simulink model "guangfu"  (R2014b)
settings: Solver=ode45  StartTime=0.0  StopTime=10.0  RelTol=1e-3
undefined symbols (not defined in the file or in its folder): K
settings Model: Creator=DELL  LastModifiedBy=dell

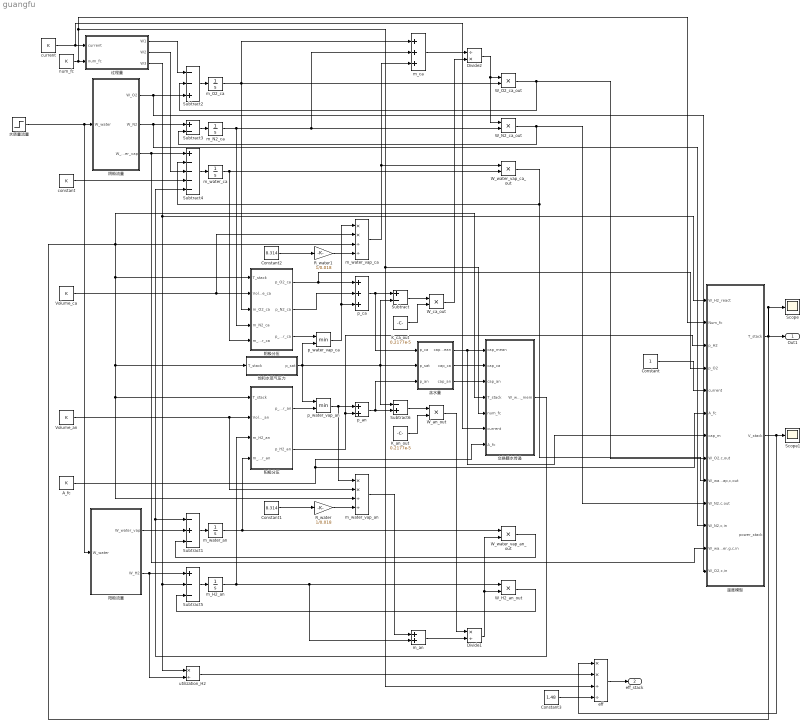
== system guangfu ==
  A_fc : Constant  Value=K
  Constant : Constant
  Constant1 : Constant  Value=8.314
  Constant2 : Constant  Value=8.314
  Constant3 : Constant  Value=1.48
  Divide1 : Product  Inputs=*/
  Divide2 : Product  Inputs=/*
  K_an_out : Constant  Value=0.2177e-5
  K_ca_out : Constant  Value=0.2177e-5
  R_water : Gain  Gain=1/0.018
  R_water1 : Gain  Gain=1/0.018
  Scope : Scope
  Scope1 : Scope
  Subtract : Sum  Inputs=+-
  Subtract1 : Sum  Inputs=-+-
  Subtract2 : Sum  Inputs=--+
  Subtract3 : Sum  Inputs=+-
  Subtract4 : Sum  Inputs=+----
  Subtract5 : Sum  Inputs=+--
  Subtract6 : Sum  Inputs=-+
  Volume_an : Constant  Value=K
  Volume_ca : Constant  Value=K
  W_H2_an_out : Product
  W_N2_ca_out : Product
  W_O2_ca_out : Product
  W_an_out : Product
  W_ca_out : Product
  W_water_vap_an_out : Product
  W_water_vap_ca_out : Product
  constant : Constant  Value=K
  current : Constant  Value=K
  eff : Product  Inputs=**//
  m_H2_an : Integrator
  m_N2_ca : Integrator
  m_O2_ca : Integrator
  m_an : Sum
  m_ca : Sum  Inputs=+++
  m_water_an : Integrator
  m_water_ca : Integrator
  m_water_vap_an : Product  Inputs=**//
  m_water_vap_ca : Product  Inputs=**//
  num_fc : Constant  Value=K
  p_an : Sum
  p_ca : Sum  Inputs=3
  p_water_vap_an : MinMax  Inputs=2
  p_water_vap_ca : MinMax  Inputs=2
  utilization_H2 : Product  Inputs=*/
  交换膜水传递 : Subsystem  TreatAsAtomicUnit=on
  含水量 : Subsystem
  水质量流量 : Step  SampleTime=0
  温度模型 : Subsystem
  过程量 : Subsystem
  阳极分压 : Subsystem
  阳极流量 : Subsystem
  阴极分压 : Subsystem
  阴极流量 : Subsystem  TreatAsAtomicUnit=on
  饱和水蒸气压力 : Subsystem
  Out1 : Outport
  eff_stack : Outport  Port=2
  wires:
  温度模型/2(V_stack) -> Scope1/1, eff/1
  Constant/1 -> 温度模型/5(current)
  Volume_ca/1 -> m_water_vap_ca/2, 阴极分压/2(Volume_ca)
  阴极分压/3(p_water_ca) -> p_water_vap_ca/1
  饱和水蒸气压力/1(p_sat) -> p_water_vap_an/1, Subtract/2, 含水量/2(p_sat), Subtract6/1, p_water_vap_ca/2
  p_water_vap_ca/1 -> m_water_vap_ca/1, p_ca/3
  p_ca/1 -> Subtract/1, 含水量/1(p_ca)
  Subtract/1 -> W_ca_out/1
  K_ca_out/1 -> W_ca_out/2
  阴极流量/1(W_O2) -> 温度模型/13(W_O2,c,in), Subtract2/3
  过程量/3(W3) -> utilization_H2/1, Subtract5/2, 温度模型/1(W_H2_react)
  过程量/1(W1) -> Subtract2/1
  Subtract2/1 -> m_O2_ca/1
  阴极流量/2(W_N2) -> 温度模型/11(W_N2,c,in), Subtract3/1
  Subtract3/1 -> m_N2_ca/1
  阴极流量/3(W_water_vap) -> 温度模型/12(W_water,g,c,in), Subtract4/1
  Subtract4/1 -> m_water_ca/1
  过程量/2(W2) -> Subtract4/3
  constant/1 -> Subtract4/4
  m_O2_ca/1 -> W_O2_ca_out/2, m_ca/1, 阴极分压/3(m_O2_ca)
  m_N2_ca/1 -> W_N2_ca_out/2, m_ca/2, 阴极分压/4(m_N2_ca)
  温度模型/1(T_stack) -> m_water_vap_an/3, 阳极分压/1(T_stack), 饱和水蒸气压力/1(T_stack), 阴极分压/1(T_stack), 交换膜水传递/4(T_stack), m_water_vap_ca/3, Scope/1, Out1/1
  m_water_vap_ca/1 -> m_ca/3, W_water_vap_ca_out/1
  m_water_ca/1 -> W_water_vap_ca_out/2, 阴极分压/5(m_water_ca)
  Constant2/1 -> R_water1/1
  R_water1/1 -> m_water_vap_ca/4
  阴极分压/2(p_N2_ca) -> p_ca/2
  m_ca/1 -> Divide2/1
  W_ca_out/1 -> Divide2/2
  Divide2/1 -> W_N2_ca_out/1, W_O2_ca_out/1
  W_O2_ca_out/1 -> 温度模型/8(W_O2,c,out), Subtract2/2
  W_N2_ca_out/1 -> 温度模型/10(W_N2,c,out), Subtract3/2
  W_water_vap_ca_out/1 -> Subtract4/2, 温度模型/9(W_water,vap,c,out)
  交换膜水传递/1(W_water_mem) -> Subtract4/5, Subtract1/1
  水质量流量/1 -> 阳极流量/1(W_water), 阴极流量/1(W_water)
  阳极流量/2(W_H2) -> utilization_H2/2, Subtract5/1
  Subtract5/1 -> m_H2_an/1
  Subtract1/1 -> m_water_an/1
  阳极分压/1(p_water_an) -> p_water_vap_an/2
  p_water_vap_an/1 -> p_an/1, m_water_vap_an/1
  阳极分压/2(p_H2_an) -> 温度模型/3(p_H2), p_an/2
  Constant1/1 -> R_water/1
  R_water/1 -> m_water_vap_an/4
  Volume_an/1 -> 阳极分压/2(Volume_an), m_water_vap_an/2
  Subtract6/1 -> W_an_out/1
  K_an_out/1 -> W_an_out/2
  m_water_vap_an/1 -> m_an/1
  m_H2_an/1 -> 阳极分压/3(m_H2_an), W_H2_an_out/1, m_an/2
  W_an_out/1 -> Divide1/1
  m_an/1 -> Divide1/2
  m_water_an/1 -> 阳极分压/4(m_water_an), W_water_vap_an_out/1
  Divide1/1 -> W_H2_an_out/2, W_water_vap_an_out/2
  阳极流量/1(W_water_vap) -> Subtract1/2
  W_water_vap_an_out/1 -> Subtract1/3
  W_H2_an_out/1 -> Subtract5/3
  p_an/1 -> Subtract6/2, 含水量/3(p_an)
  含水量/1(cap_mean) -> 温度模型/7(cap_m), 交换膜水传递/1(cap_mean)
  current/1 -> 交换膜水传递/6(current), 过程量/1(current)
  含水量/2(cap_ca) -> 交换膜水传递/2(cap_ca)
  含水量/3(cap_an) -> 交换膜水传递/3(cap_an)
  A_fc/1 -> 温度模型/6(A_fc), 交换膜水传递/7(A_fc)
  utilization_H2/1 -> eff/2
  num_fc/1 -> 温度模型/2(Num_fc), eff/3, 交换膜水传递/5(num_fc), 过程量/2(num_fc)
  Constant3/1 -> eff/4
  eff/1 -> eff_stack/1
  阴极分压/1(p_O2_ca) -> 温度模型/4(p_O2), p_ca/1

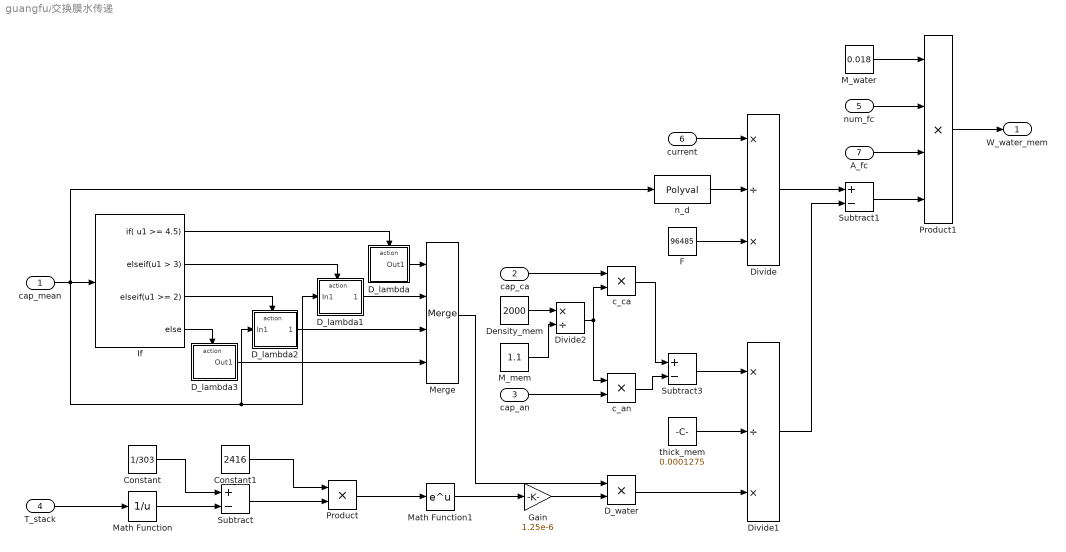
== system guangfu/交换膜水传递 ==
  cap_mean : Inport
  cap_ca : Inport  Port=2
  cap_an : Inport  Port=3
  T_stack : Inport  Port=4
  num_fc : Inport  Port=5
  current : Inport  Port=6
  A_fc : Inport  Port=7
  Constant : Constant  Value=1/303
  Constant1 : Constant  Value=2416
  D_lambda : Subsystem  TreatAsAtomicUnit=on
  D_lambda1 : Subsystem  TreatAsAtomicUnit=on
  D_lambda2 : Subsystem  TreatAsAtomicUnit=on
  D_lambda3 : Subsystem  TreatAsAtomicUnit=on
  D_water : Product
  Density_mem : Constant  Value=2000
  Divide : Product  Inputs=*/*
  Divide1 : Product  Inputs=*/*
  Divide2 : Product  Inputs=*/
  F : Constant  Value=96485
  Gain : Gain  Gain=1.25e-6
  If : If  IfExpression=u1 >= 4.5  ElseIfExpressions=u1 > 3,u1 >= 2  ZeroCross=off
  M_mem : Constant  Value=1.1
  M_water : Constant  Value=0.018
  Math Function : Math  Operator=reciprocal  SaturateOnIntegerOverflow=on
  Math Function1 : Math  SaturateOnIntegerOverflow=on
  Merge : Merge  Inputs=4
  Product : Product
  Product1 : Product  Inputs=4
  Subtract : Sum  Inputs=+-
  Subtract1 : Sum  Inputs=+-
  Subtract3 : Sum  Inputs=+-
  c_an : Product
  c_ca : Product
  n_d : Polyval  Coefs=[0.0029,0.05,-3.4e-19]
  thick_mem : Constant  Value=0.0001275
  W_water_mem : Outport
  wires:
  If/1 -> D_lambda/Action
  If/2 -> D_lambda1/Action
  If/3 -> D_lambda2/Action
  If/4 -> D_lambda3/Action
  D_lambda/1(Out1) -> Merge/1
  D_lambda1/1(Out1) -> Merge/2
  D_lambda2/1(Out1) -> Merge/3
  D_lambda3/1(Out1) -> Merge/4
  T_stack/1 -> Math Function/1
  Math Function/1 -> Subtract/2
  Constant/1 -> Subtract/1
  Subtract/1 -> Product/2
  Constant1/1 -> Product/1
  Product/1 -> Math Function1/1
  Math Function1/1 -> Gain/1
  Merge/1 -> D_water/1
  cap_mean/1 -> n_d/1, D_lambda1/1(In1), D_lambda2/1(In1), If/1
  n_d/1 -> Divide/2
  F/1 -> Divide/3
  current/1 -> Divide/1
  cap_ca/1 -> c_ca/1
  Divide/1 -> Subtract1/1
  Divide1/1 -> Subtract1/2
  D_water/1 -> Divide1/3
  thick_mem/1 -> Divide1/2
  Subtract3/1 -> Divide1/1
  Subtract1/1 -> Product1/4
  A_fc/1 -> Product1/3
  num_fc/1 -> Product1/2
  M_water/1 -> Product1/1
  Product1/1 -> W_water_mem/1
  M_mem/1 -> Divide2/2
  Density_mem/1 -> Divide2/1
  Divide2/1 -> c_an/1, c_ca/2
  c_an/1 -> Subtract3/2
  c_ca/1 -> Subtract3/1
  cap_an/1 -> c_an/2
  Gain/1 -> D_water/2

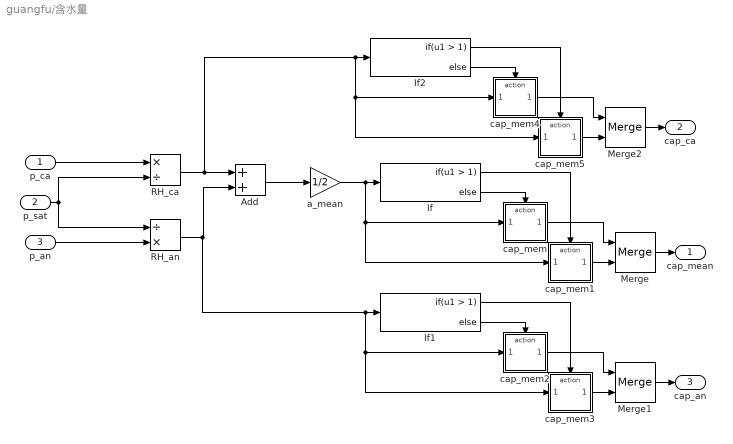
== system guangfu/含水量 ==
  p_ca : Inport
  p_sat : Inport  Port=2
  p_an : Inport  Port=3
  Add : Sum
  If : If  IfExpression=u1 > 1
  If1 : If  IfExpression=u1 > 1
  If2 : If  IfExpression=u1 > 1
  Merge : Merge
  Merge1 : Merge
  Merge2 : Merge
  RH_an : Product  Inputs=/*
  RH_ca : Product  Inputs=*/
  a_mean : Gain  Gain=1/2
  cap_mem : Subsystem  TreatAsAtomicUnit=on
  cap_mem1 : Subsystem  TreatAsAtomicUnit=on
  cap_mem2 : Subsystem  TreatAsAtomicUnit=on
  cap_mem3 : Subsystem  TreatAsAtomicUnit=on
  cap_mem4 : Subsystem  TreatAsAtomicUnit=on
  cap_mem5 : Subsystem  TreatAsAtomicUnit=on
  cap_mean : Outport
  cap_ca : Outport  Port=2
  cap_an : Outport  Port=3
  wires:
  Add/1 -> a_mean/1
  cap_mem/1(Out1) -> Merge/1
  a_mean/1 -> cap_mem1/1(In1), cap_mem/1(In1), If/1
  Merge/1 -> cap_mean/1
  If/2 -> cap_mem/Action
  p_ca/1 -> RH_ca/1
  cap_mem1/1(Out1) -> Merge/2
  If/1 -> cap_mem1/Action
  p_sat/1 -> RH_ca/2, RH_an/1
  p_an/1 -> RH_an/2
  cap_mem2/1(Out1) -> Merge1/1
  RH_an/1 -> cap_mem3/1(In1), cap_mem2/1(In1), If1/1, Add/2
  Merge1/1 -> cap_an/1
  If1/2 -> cap_mem2/Action
  cap_mem3/1(Out1) -> Merge1/2
  If1/1 -> cap_mem3/Action
  cap_mem4/1(Out1) -> Merge2/1
  RH_ca/1 -> cap_mem5/1(In1), cap_mem4/1(In1), If2/1, Add/1
  Merge2/1 -> cap_ca/1
  If2/2 -> cap_mem4/Action
  cap_mem5/1(Out1) -> Merge2/2
  If2/1 -> cap_mem5/Action

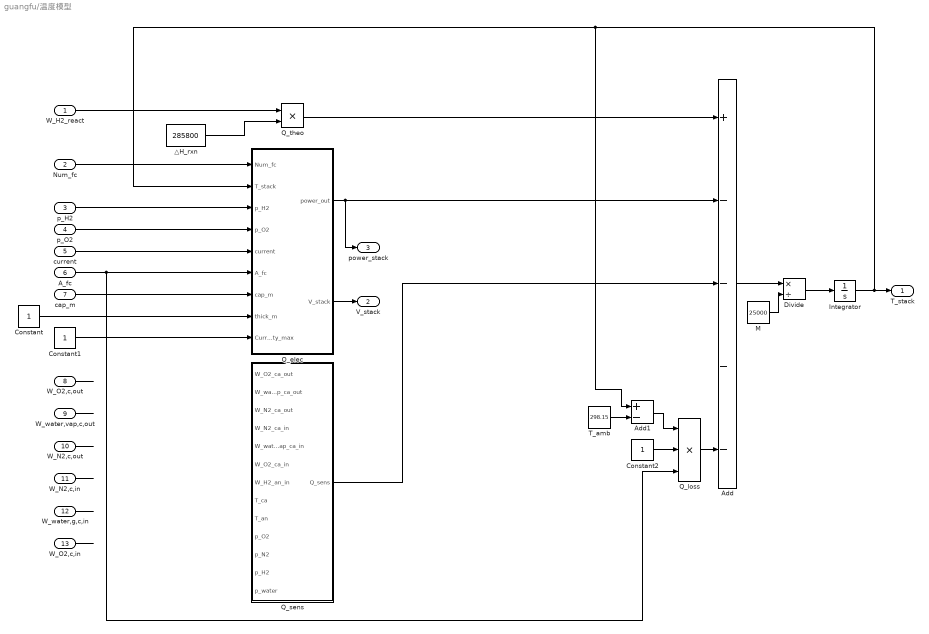
== system guangfu/温度模型 ==
  W_H2_react : Inport
  Num_fc : Inport  Port=2
  p_H2 : Inport  Port=3
  p_O2 : Inport  Port=4
  current : Inport  Port=5
  A_fc : Inport  Port=6
  cap_m : Inport  Port=7
  W_O2,c,out : Inport  Port=8
  W_water,vap,c,out : Inport  Port=9
  W_N2,c,out : Inport  Port=10
  W_N2,c,in : Inport  Port=11
  W_water,g,c,in : Inport  Port=12
  W_O2,c,in : Inport  Port=13
  Add : Sum  Inputs=+----
  Add1 : Sum  Inputs=+-
  Constant : Constant
  Constant1 : Constant
  Constant2 : Constant
  Divide : Product  Inputs=*/
  Integrator : Integrator
  M : Constant  Value=25000
  Q_elec : Subsystem
  Q_loss : Product  Inputs=3
  Q_sens : Subsystem
  Q_theo : Product
  T_amb : Constant  Value=298.15
  △H_rxn : Constant  Value=285800
  T_stack : Outport
  V_stack : Outport  Port=2
  power_stack : Outport  Port=3
  wires:
  W_H2_react/1 -> Q_theo/1
  current/1 -> Q_elec/5(current)
  p_O2/1 -> Q_elec/4(p_O2)
  p_H2/1 -> Q_elec/3(p_H2)
  W_O2,c,out/1 -> ?
  W_water,vap,c,out/1 -> ?
  W_N2,c,out/1 -> ?
  W_N2,c,in/1 -> ?
  W_water,g,c,in/1 -> ?
  W_O2,c,in/1 -> ?
  Q_elec/2(V_stack) -> V_stack/1
  △H_rxn/1 -> Q_theo/2
  Q_elec/1(power_out) -> Add/2, power_stack/1
  Q_theo/1 -> Add/1
  Q_sens/1(Q_sens) -> Add/3
  Add/1 -> Divide/1
  M/1 -> Divide/2
  Add1/1 -> Q_loss/1
  Q_loss/1 -> Add/5
  Constant2/1 -> Q_loss/2
  Divide/1 -> Integrator/1
  Integrator/1 -> Add1/1, Q_elec/2(T_stack), T_stack/1
  Num_fc/1 -> Q_elec/1(Num_fc)
  cap_m/1 -> Q_elec/7(cap_m)
  Constant/1 -> Q_elec/8(thick_m)
  T_amb/1 -> Add1/2
  A_fc/1 -> Q_loss/3, Q_elec/6(A_fc)
  Constant1/1 -> Q_elec/9(CurrentDensity_max)

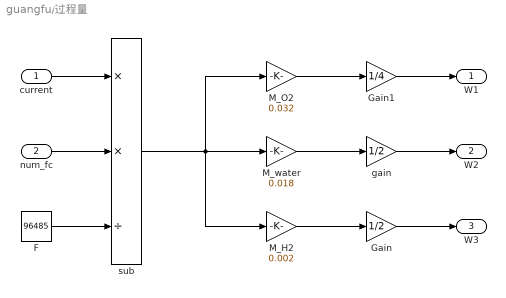
== system guangfu/过程量 ==
  current : Inport
  num_fc : Inport  Port=2
  F : Constant  Value=96485
  Gain : Gain  Gain=1/2
  Gain1 : Gain  Gain=1/4
  M_H2 : Gain  Gain=0.002
  M_O2 : Gain  Gain=0.032
  M_water : Gain  Gain=0.018
  gain : Gain  Gain=1/2
  sub : Product  Inputs=**/
  W1 : Outport
  W2 : Outport  Port=2
  W3 : Outport  Port=3
  wires:
  current/1 -> sub/1
  sub/1 -> M_water/1, M_O2/1, M_H2/1
  num_fc/1 -> sub/2
  F/1 -> sub/3
  M_H2/1 -> Gain/1
  Gain1/1 -> W1/1
  M_O2/1 -> Gain1/1
  Gain/1 -> W3/1
  M_water/1 -> gain/1
  gain/1 -> W2/1

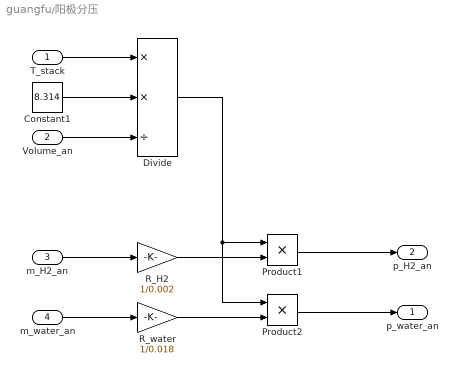
== system guangfu/阳极分压 ==
  T_stack : Inport
  Volume_an : Inport  Port=2
  m_H2_an : Inport  Port=3
  m_water_an : Inport  Port=4
  Constant1 : Constant  Value=8.314
  Divide : Product  Inputs=**/
  Product1 : Product
  Product2 : Product
  R_H2 : Gain  Gain=1/0.002
  R_water : Gain  Gain=1/0.018
  p_water_an : Outport
  p_H2_an : Outport  Port=2
  wires:
  T_stack/1 -> Divide/1
  Volume_an/1 -> Divide/3
  Constant1/1 -> Divide/2
  m_H2_an/1 -> R_H2/1
  m_water_an/1 -> R_water/1
  R_H2/1 -> Product1/2
  R_water/1 -> Product2/2
  Product1/1 -> p_H2_an/1
  Product2/1 -> p_water_an/1
  Divide/1 -> Product2/1, Product1/1

== system guangfu/阳极流量 ==
  W_water : Inport
  Constant1 : Constant
  Constant2 : Constant
  W_H2_in : Product
  W_water_in : Product
  x_H2 : Sum  Inputs=+-
  W_water_vap : Outport
  W_H2 : Outport  Port=2
  wires:
  W_water/1 -> W_water_in/1, W_H2_in/1
  ? -> W_water_in/2, x_H2/2
  Constant1/1 -> x_H2/1
  x_H2/1 -> W_H2_in/2
  W_H2_in/1 -> W_H2/1
  W_water_in/1 -> W_water_vap/1

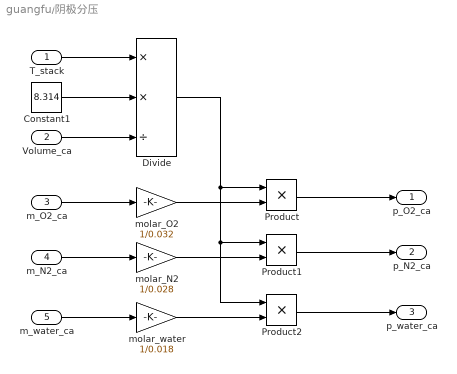
== system guangfu/阴极分压 ==
  T_stack : Inport
  Volume_ca : Inport  Port=2
  m_O2_ca : Inport  Port=3
  m_N2_ca : Inport  Port=4
  m_water_ca : Inport  Port=5
  Constant1 : Constant  Value=8.314
  Divide : Product  Inputs=**/
  Product : Product
  Product1 : Product
  Product2 : Product
  molar_N2 : Gain  Gain=1/0.028
  molar_O2 : Gain  Gain=1/0.032
  molar_water : Gain  Gain=1/0.018
  p_O2_ca : Outport
  p_N2_ca : Outport  Port=2
  p_water_ca : Outport  Port=3
  wires:
  T_stack/1 -> Divide/1
  Volume_ca/1 -> Divide/3
  Constant1/1 -> Divide/2
  m_O2_ca/1 -> molar_O2/1
  m_N2_ca/1 -> molar_N2/1
  m_water_ca/1 -> molar_water/1
  molar_O2/1 -> Product/2
  Divide/1 -> Product/1, Product1/1, Product2/1
  Product/1 -> p_O2_ca/1
  molar_N2/1 -> Product1/2
  molar_water/1 -> Product2/2
  Product1/1 -> p_N2_ca/1
  Product2/1 -> p_water_ca/1

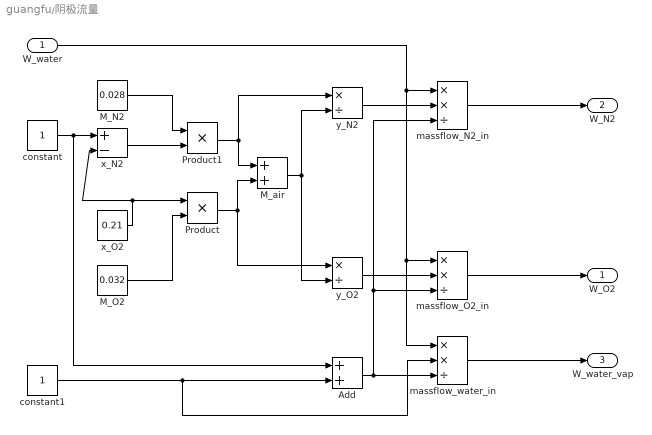
== system guangfu/阴极流量 ==
  W_water : Inport
  Add : Sum
  M_N2 : Constant  Value=0.028
  M_O2 : Constant  Value=0.032
  M_air : Sum
  Product : Product
  Product1 : Product
  constant : Constant
  constant1 : Constant
  massflow_N2_in : Product  Inputs=**/
  massflow_O2_in : Product  Inputs=**/
  massflow_water_in : Product  Inputs=**/
  x_N2 : Sum  Inputs=+-
  x_O2 : Constant  Value=0.21
  y_N2 : Product  Inputs=*/
  y_O2 : Product  Inputs=*/
  W_O2 : Outport
  W_N2 : Outport  Port=2
  W_water_vap : Outport  Port=3
  wires:
  constant/1 -> Add/1, x_N2/1
  x_O2/1 -> Product/1, x_N2/2
  M_O2/1 -> Product/2
  M_N2/1 -> Product1/1
  x_N2/1 -> Product1/2
  Product1/1 -> M_air/1, y_N2/1
  Product/1 -> M_air/2, y_O2/1
  M_air/1 -> y_O2/2, y_N2/2
  constant1/1 -> massflow_water_in/2, Add/2
  W_water/1 -> massflow_water_in/1, massflow_O2_in/1, massflow_N2_in/1
  y_N2/1 -> massflow_N2_in/2
  Add/1 -> massflow_water_in/3, massflow_N2_in/3, massflow_O2_in/3
  y_O2/1 -> massflow_O2_in/2
  massflow_N2_in/1 -> W_N2/1
  massflow_O2_in/1 -> W_O2/1
  massflow_water_in/1 -> W_water_vap/1

== system guangfu/饱和水蒸气压力 ==
  T_stack : Inport
  Constant : Constant  Value=273.15
  Math Function : Math  Operator=10^u  SaturateOnIntegerOverflow=on
  Polynomial : Polyval  Coefs=[1.4454e-7,-9.1837e-5,0.2953,-2.1794]
  T : Sum  Inputs=+-
  p_sat : Outport
  wires:
  Polynomial/1 -> Math Function/1
  T_stack/1 -> T/1
  Math Function/1 -> p_sat/1
  T/1 -> Polynomial/1
  Constant/1 -> T/2

== system guangfu/交换膜水传递/D_lambda ==
  Action Port : ActionPort  ActionType=then
  Constant : Constant  Value=1.25e-6
  Out1 : Outport
  wires:
  Constant/1 -> Out1/1

== system guangfu/交换膜水传递/D_lambda1 ==
  In1 : Inport
  Action Port : ActionPort  ActionType=elseif
  Constant : Constant  Value=3
  Constant1 : Constant  Value=1.67
  Gain : Gain  Gain=1e-6
  Product : Product
  Subtract : Sum  Inputs=+-
  Subtract1 : Sum  Inputs=+-
  Out1 : Outport
  wires:
  In1/1 -> Subtract/1
  Constant/1 -> Subtract/2, Subtract1/1
  Constant1/1 -> Product/1
  Subtract/1 -> Product/2
  Product/1 -> Subtract1/2
  Subtract1/1 -> Gain/1
  Gain/1 -> Out1/1

== system guangfu/交换膜水传递/D_lambda2 ==
  In1 : Inport
  Action Port : ActionPort  ActionType=elseif
  Add : Sum
  Constant : Constant  Value=2
  Constant1 : Constant
  Gain : Gain  Gain=1e-6
  Product : Product
  Subtract : Sum  Inputs=+-
  Out1 : Outport
  wires:
  In1/1 -> Subtract/1
  Constant/1 -> Product/2, Subtract/2
  Subtract/1 -> Product/1
  Product/1 -> Add/2
  Add/1 -> Gain/1
  Gain/1 -> Out1/1
  Constant1/1 -> Add/1

== system guangfu/交换膜水传递/D_lambda3 ==
  Action Port : ActionPort  ActionType=else
  Constant : Constant  Value=1e-6
  Out1 : Outport
  wires:
  Constant/1 -> Out1/1

== system guangfu/含水量/cap_mem ==
  In1 : Inport
  Action Port : ActionPort  ActionType=else
  Polynomial : Polyval  Coefs=[36,-39.85,17.81,0.043]
  Out1 : Outport
  wires:
  In1/1 -> Polynomial/1
  Polynomial/1 -> Out1/1

== system guangfu/含水量/cap_mem1 ==
  In1 : Inport
  Action Port : ActionPort  ActionType=then
  Polynomial : Polyval  Coefs=[1.4,-14]
  Out1 : Outport
  wires:
  In1/1 -> Polynomial/1
  Polynomial/1 -> Out1/1

== system guangfu/含水量/cap_mem2 ==
  In1 : Inport
  Action Port : ActionPort  ActionType=else
  Polynomial : Polyval  Coefs=[36,-39.85,17.81,0.043]
  Out1 : Outport
  wires:
  In1/1 -> Polynomial/1
  Polynomial/1 -> Out1/1

== system guangfu/含水量/cap_mem3 ==
  In1 : Inport
  Action Port : ActionPort  ActionType=then
  Polynomial : Polyval  Coefs=[1.4,-14]
  Out1 : Outport
  wires:
  In1/1 -> Polynomial/1
  Polynomial/1 -> Out1/1

== system guangfu/含水量/cap_mem4 ==
  In1 : Inport
  Action Port : ActionPort  ActionType=else
  Polynomial : Polyval  Coefs=[36,-39.85,17.81,0.043]
  Out1 : Outport
  wires:
  In1/1 -> Polynomial/1
  Polynomial/1 -> Out1/1

== system guangfu/含水量/cap_mem5 ==
  In1 : Inport
  Action Port : ActionPort  ActionType=then
  Polynomial : Polyval  Coefs=[1.4,-14]
  Out1 : Outport
  wires:
  In1/1 -> Polynomial/1
  Polynomial/1 -> Out1/1

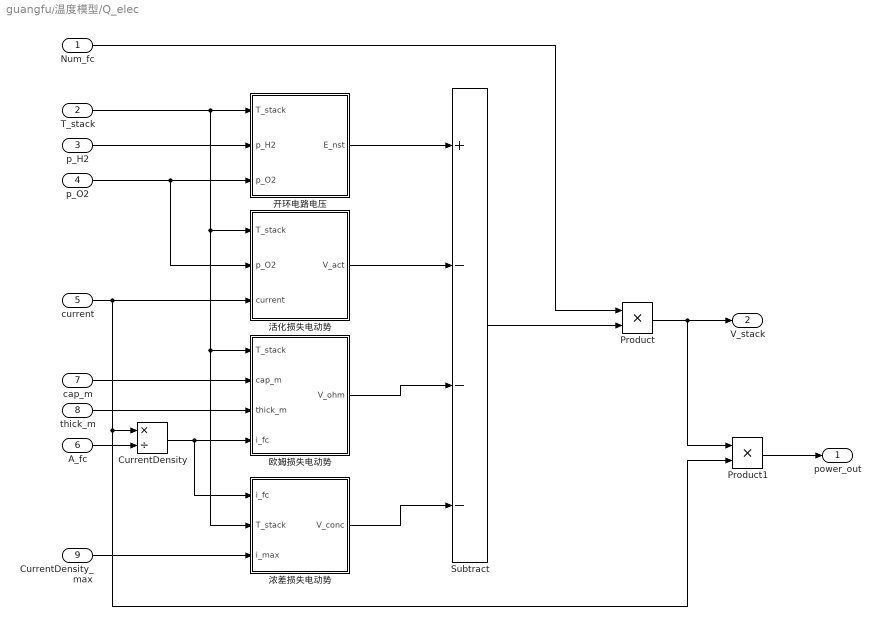
== system guangfu/温度模型/Q_elec ==
  Num_fc : Inport
  T_stack : Inport  Port=2
  p_H2 : Inport  Port=3
  p_O2 : Inport  Port=4
  current : Inport  Port=5
  A_fc : Inport  Port=6
  cap_m : Inport  Port=7
  thick_m : Inport  Port=8
  CurrentDensity_max : Inport  Port=9
  CurrentDensity : Product  Inputs=*/
  Product : Product
  Product1 : Product
  Subtract : Sum  Inputs=+---
  开环电路电压 : Subsystem  TreatAsAtomicUnit=on
  欧姆损失电动势 : MATLAB Function  TreatAsAtomicUnit=on
  活化损失电动势 : MATLAB Function  TreatAsAtomicUnit=on
  浓差损失电动势 : Subsystem
  power_out : Outport
  V_stack : Outport  Port=2
  wires:
  p_H2/1 -> 开环电路电压/2(p_H2)
  p_O2/1 -> 活化损失电动势/2(p_O2), 开环电路电压/3(p_O2)
  T_stack/1 -> 开环电路电压/1(T_stack), 浓差损失电动势/2(T_stack), 欧姆损失电动势/1(T_stack), 活化损失电动势/1(T_stack)
  current/1 -> Product1/2, CurrentDensity/1, 活化损失电动势/3(current)
  cap_m/1 -> 欧姆损失电动势/2(cap_m)
  开环电路电压/1(E_nst) -> Subtract/1
  活化损失电动势/1(V_act) -> Subtract/2
  欧姆损失电动势/1(V_ohm) -> Subtract/3
  浓差损失电动势/1(V_conc) -> Subtract/4
  Subtract/1 -> Product/2
  Product/1 -> Product1/1, V_stack/1
  Product1/1 -> power_out/1
  Num_fc/1 -> Product/1
  thick_m/1 -> 欧姆损失电动势/3(thick_m)
  A_fc/1 -> CurrentDensity/2
  CurrentDensity/1 -> 浓差损失电动势/1(i_fc), 欧姆损失电动势/4(i_fc)
  CurrentDensity_max/1 -> 浓差损失电动势/3(i_max)

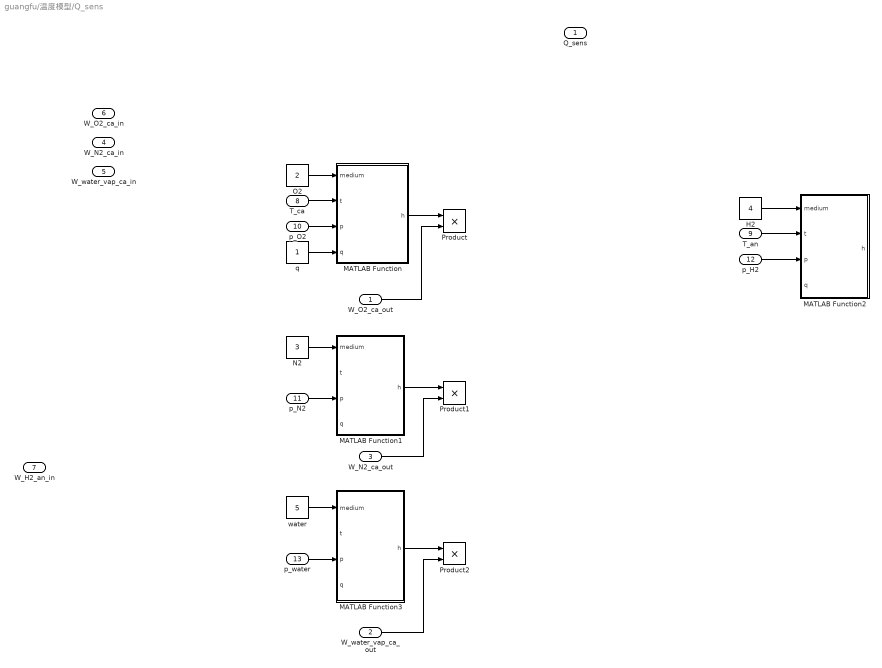
== system guangfu/温度模型/Q_sens ==
  W_O2_ca_out : Inport
  W_water_vap_ca_out : Inport  Port=2
  W_N2_ca_out : Inport  Port=3
  W_N2_ca_in : Inport  Port=4
  W_water_vap_ca_in : Inport  Port=5
  W_O2_ca_in : Inport  Port=6
  W_H2_an_in : Inport  Port=7
  T_ca : Inport  Port=8
  T_an : Inport  Port=9
  p_O2 : Inport  Port=10
  p_N2 : Inport  Port=11
  p_H2 : Inport  Port=12
  p_water : Inport  Port=13
  H2 : Constant  Value=4
  MATLAB Function : MATLAB Function  TreatAsAtomicUnit=on
  MATLAB Function1 : MATLAB Function  TreatAsAtomicUnit=on
  MATLAB Function2 : MATLAB Function  TreatAsAtomicUnit=on
  MATLAB Function3 : MATLAB Function  TreatAsAtomicUnit=on
  N2 : Constant  Value=3
  O2 : Constant  Value=2
  Product : Product
  Product1 : Product
  Product2 : Product
  q : Constant
  water : Constant  Value=5
  Q_sens : Outport
  wires:
  W_O2_ca_out/1 -> Product/2
  O2/1 -> MATLAB Function/1(medium)
  N2/1 -> MATLAB Function1/1(medium)
  H2/1 -> MATLAB Function2/1(medium)
  water/1 -> MATLAB Function3/1(medium)
  T_ca/1 -> MATLAB Function/2(t)
  p_O2/1 -> MATLAB Function/3(p)
  p_N2/1 -> MATLAB Function1/3(p)
  p_H2/1 -> MATLAB Function2/3(p)
  T_an/1 -> MATLAB Function2/2(t)
  p_water/1 -> MATLAB Function3/3(p)
  q/1 -> MATLAB Function/4(q)
  MATLAB Function/1(h) -> Product/1
  MATLAB Function1/1(h) -> Product1/1
  W_N2_ca_out/1 -> Product1/2
  MATLAB Function3/1(h) -> Product2/1
  W_water_vap_ca_out/1 -> Product2/2

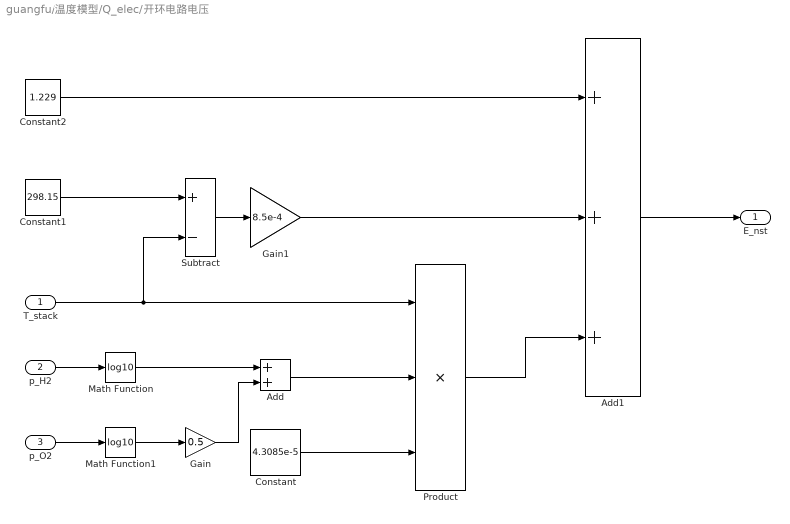
== system guangfu/温度模型/Q_elec/开环电路电压 ==
  T_stack : Inport
  p_H2 : Inport  Port=2
  p_O2 : Inport  Port=3
  Add : Sum
  Add1 : Sum  Inputs=+++
  Constant : Constant  Value=4.3085e-5
  Constant1 : Constant  Value=298.15
  Constant2 : Constant  Value=1.229
  Gain : Gain  Gain=0.5
  Gain1 : Gain  Gain=8.5e-4
  Math Function : Math  Operator=log10  SaturateOnIntegerOverflow=on
  Math Function1 : Math  Operator=log10  SaturateOnIntegerOverflow=on
  Product : Product  Inputs=3
  Subtract : Sum  Inputs=+-
  E_nst : Outport
  wires:
  p_H2/1 -> Math Function/1
  p_O2/1 -> Math Function1/1
  Math Function1/1 -> Gain/1
  Gain/1 -> Add/2
  Math Function/1 -> Add/1
  T_stack/1 -> Subtract/2, Product/1
  Add/1 -> Product/2
  Constant/1 -> Product/3
  Constant1/1 -> Subtract/1
  Subtract/1 -> Gain1/1
  Constant2/1 -> Add1/1
  Gain1/1 -> Add1/2
  Product/1 -> Add1/3
  Add1/1 -> E_nst/1

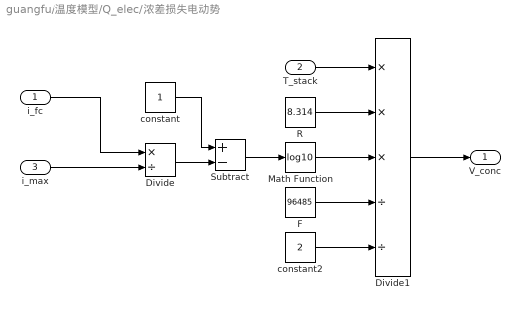
== system guangfu/温度模型/Q_elec/浓差损失电动势 ==
  i_fc : Inport
  T_stack : Inport  Port=2
  i_max : Inport  Port=3
  Divide : Product  Inputs=*/
  Divide1 : Product  Inputs=***//
  F : Constant  Value=96485
  Math Function : Math  Operator=log10  SaturateOnIntegerOverflow=on
  R : Constant  Value=8.314
  Subtract : Sum  Inputs=+-
  constant : Constant
  constant2 : Constant  Value=2
  V_conc : Outport
  wires:
  i_fc/1 -> Divide/1
  i_max/1 -> Divide/2
  constant/1 -> Subtract/1
  Divide/1 -> Subtract/2
  Divide1/1 -> V_conc/1
  Subtract/1 -> Math Function/1
  Math Function/1 -> Divide1/3
  R/1 -> Divide1/2
  T_stack/1 -> Divide1/1
  F/1 -> Divide1/4
  constant2/1 -> Divide1/5

== matlab function guangfu/温度模型/Q_elec/欧姆损失电动势 ==
  data: T_stack input; V_ohm output; cap_m input; thick_m input; i_fc input
function V_ohm = fcn( T_stack,cap_m,thick_m,i_fc )
b1=0.005139*cap_m-0.00326;
b2=1286;
cond_m=b1*exp(b2*(1/303-1/T_stack));
R_ohm=thick_m/cond_m;
V_ohm=i_fc*R_ohm;

== matlab function guangfu/温度模型/Q_elec/活化损失电动势 ==
  data: T_stack input; V_act output; p_O2 input; current input
function V_act = fcn( T_stack,p_O2,current )
%#codegen
V_act=0.9514-3.12e-3*T_stack+1.87e-4*T_stack*ln(current)-7.4e-5*T_stack*ln(p_O2/(5.08e6*exp(-498/T_stack)));

== matlab function guangfu/温度模型/Q_sens/MATLAB Function ==
  data: medium input; t input; p input; q input; h output
function h = fcn(medium,t,p,q)
%#codegen
rho=1;
cv=1;
cp=1;
h=1;
k=1;
mu=1;
coder.extrinsic('props');
[ rho,cv,cp,h,mu,k ] = props( medium,t,p,q );

== matlab function guangfu/温度模型/Q_sens/MATLAB Function1 ==
  data: medium input; t input; p input; q input; h output
function h = fcn(medium,t,p,q)
%#codegen
rho=1;
cv=1;
cp=1;
h=1;
k=1;
mu=1;
coder.extrinsic('props');
[ rho,cv,cp,h,mu,k ] = props( medium,t,p,q );

== matlab function guangfu/温度模型/Q_sens/MATLAB Function2 ==
  data: medium input; t input; p input; q input; h output
function h = fcn(medium,t,p,q)
%#codegen
rho=1;
cv=1;
cp=1;
h=1;
k=1;
mu=1;
coder.extrinsic('props');
[ rho,cv,cp,h,mu,k ] = props( medium,t,p,q );

== matlab function guangfu/温度模型/Q_sens/MATLAB Function3 ==
  data: medium input; t input; p input; q input; h output
function h = fcn(medium,t,p,q)
%#codegen
rho=1;
cv=1;
cp=1;
h=1;
k=1;
mu=1;
coder.extrinsic('props');
[ rho,cv,cp,h,mu,k ] = props( medium,t,p,q );
